simulink model "le2_simu"  (R2022b)
settings: Solver=VariableStepAuto  StartTime=0.0  StopTime=180  RelTol=1e-3
settings Model: Creator=PJ  LastModifiedBy=PJ
settings DataIOCC: ReturnWorkspaceOutputs=off

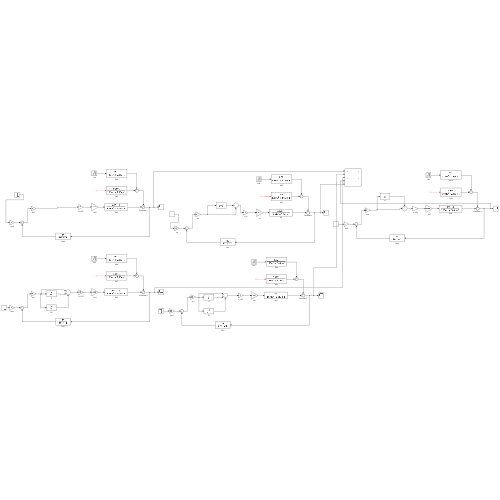
[thumbnail: Simulink's stored preview of the top-level diagram]
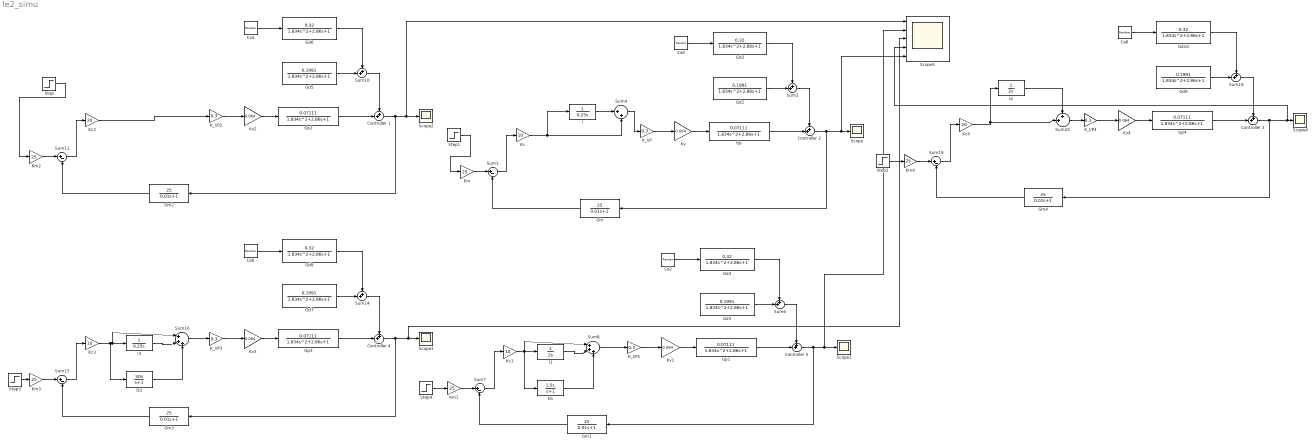
== system le2_simu ==
  Ca{0,2,4,6,8} (5 alike) : RandomNumber  Variance=0.01  Seed=1  SampleTime=0.1
  Controller {1..5} (5 alike) : Sum  Inputs=++|
  D1 : TransferFcn  Numerator=[1.5 0]  Denominator=[1 1]
  D3 : TransferFcn  Numerator=[50 0]  Denominator=[1 1]
  Gd{1,3,5,7,9} (5 alike) : TransferFcn  Numerator=[0.1991]  Denominator=[1.834 2.86 1]
  Gd{2,4,6,8,10} (5 alike) : TransferFcn  Numerator=[0.32]  Denominator=[1.834 2.86 1]
  Gm{,1..4} (5 alike) : TransferFcn  Numerator=[25]  Denominator=[0.01 1]  ParameterTunability=Unconstrained
  Gp{,1..4} (5 alike) : TransferFcn  Numerator=[0.07111]  Denominator=[1.834 2.86 1]
  I : TransferFcn  Denominator=[0.25 0]
  I1 : TransferFcn  Denominator=[2 0]
  I3 : TransferFcn  Denominator=[0.25 0]
  I4 : TransferFcn  Denominator=[2 0]
  K_I/P{,1..4} (5 alike) : Gain  Gain=0.3
  Kc : Gain  Gain=10
  Kc1 : Gain  Gain=10
  Kc2 : Gain  Gain=20
  Kc3 : Gain  Gain=10
  Kc4 : Gain  Gain=20
  Km{,1..4} (5 alike) : Gain  Gain=25
  Kv{,1..4} (5 alike) : Gain  Gain=0.064
  Scope{,1..4} (5 alike) : Scope
  Scope5 : Scope  NumInputPorts=5
  Step{,1..4} (5 alike) : Step  Time=60  After=-1  SampleTime=0
  Sum{2,6,10,14,18,20} (6 alike) : Sum  Inputs=++|
  Sum{3,7,11,15,19} (5 alike) : Sum  Inputs=|+-
  Sum16 : Sum  Inputs=|+++
  Sum4 : Sum  Inputs=|++
  Sum8 : Sum  Inputs=|+++
  wires:
  Km/1 -> Sum3/1
  Sum3/1 -> Kc/1
  Gm/1 -> Sum3/2
  K_I/P/1 -> Kv/1
  Kv/1 -> Gp/1
  Gp/1 -> Controller 2/2
  Sum2/1 -> Controller 2/1
  Gd1/1 -> Sum2/2
  Gd2/1 -> Sum2/1
  Controller 2/1 -> Scope5/5, Scope/1, Gm/1
  Ca0/1 -> Gd2/1
  ? -> Gd1/1
  ? -> Gd3/1
  Ca2/1 -> Gd4/1
  Sum6/1 -> Controller 5/1
  Gp1/1 -> Controller 5/2
  Gd3/1 -> Sum6/2
  Controller 5/1 -> Scope5/2, Scope1/1, Gm1/1
  Kv1/1 -> Gp1/1
  I1/1 -> Sum8/2
  Gm1/1 -> Sum7/2
  K_I/P1/1 -> Kv1/1
  Sum7/1 -> Kc1/1
  Gd4/1 -> Sum6/1
  Km1/1 -> Sum7/1
  D1/1 -> Sum8/3
  Kc2/1 -> K_I/P2/1
  ? -> Gd5/1
  Ca4/1 -> Gd6/1
  Sum10/1 -> Controller 1/1
  Gp2/1 -> Controller 1/2
  Gd5/1 -> Sum10/2
  Controller 1/1 -> Scope5/1, Scope2/1, Gm2/1
  Kv2/1 -> Gp2/1
  Gm2/1 -> Sum11/2
  K_I/P2/1 -> Kv2/1
  Sum11/1 -> Kc2/1
  Gd6/1 -> Sum10/1
  Km2/1 -> Sum11/1
  ? -> Gd7/1
  Ca6/1 -> Gd8/1
  Sum14/1 -> Controller 4/1
  Gp3/1 -> Controller 4/2
  Gd7/1 -> Sum14/2
  Controller 4/1 -> Scope5/3, Scope3/1, Gm3/1
  Kv3/1 -> Gp3/1
  I3/1 -> Sum16/2
  Gm3/1 -> Sum15/2
  K_I/P3/1 -> Kv3/1
  Sum15/1 -> Kc3/1
  Gd8/1 -> Sum14/1
  Km3/1 -> Sum15/1
  D3/1 -> Sum16/3
  ? -> Gd9/1
  Ca8/1 -> Gd10/1
  Sum18/1 -> Controller 3/1
  Gp4/1 -> Controller 3/2
  Gd9/1 -> Sum18/2
  Controller 3/1 -> Scope5/4, Scope4/1, Gm4/1
  Kv4/1 -> Gp4/1
  Gm4/1 -> Sum19/2
  K_I/P4/1 -> Kv4/1
  Sum19/1 -> Kc4/1
  Gd10/1 -> Sum18/1
  Km4/1 -> Sum19/1
  Kc/1 -> Sum4/2, I/1
  I/1 -> Sum4/1
  Sum4/1 -> K_I/P/1
  I4/1 -> Sum20/1
  Kc4/1 -> I4/1, Sum20/2
  Sum20/1 -> K_I/P4/1
  Kc3/1 -> D3/1, I3/1, Sum16/1
  Sum16/1 -> K_I/P3/1
  Kc1/1 -> Sum8/1, D1/1, I1/1
  Sum8/1 -> K_I/P1/1
  Step/1 -> Km2/1
  Step1/1 -> Km/1
  Step2/1 -> Km4/1
  Step3/1 -> Km3/1
  Step4/1 -> Km1/1
